simulink model "Cinematica_Inversa (1)"  (R2019a)
settings: Solver=VariableStepAuto  StartTime=0.0  StopTime=10.0  RelTol=1e-3
libraries: arduinolib x6
settings Model: Creator=PATRICIA PEÑALOZA  LastModifiedBy=PATRICIA PEÑALOZA

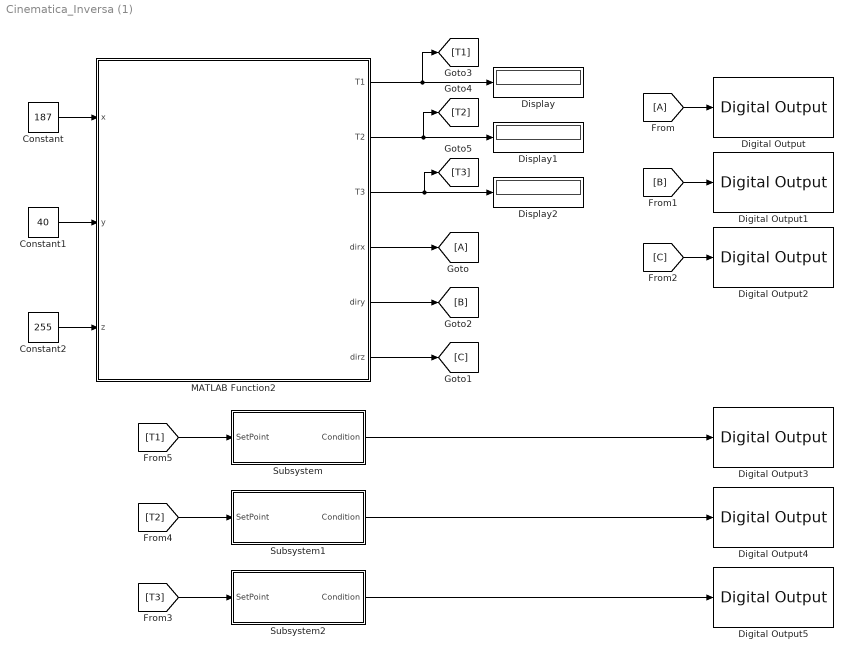
== system Cinematica_Inversa (1) ==
  Constant : Constant  Value=187
  Constant1 : Constant  Value=40
  Constant2 : Constant  Value=255
  Digital Output{,1..5} (6 alike) : arduinolib/Digital Output  pinNumber=9  blockPlatform=arduino
  Display : Display
  Display1 : Display
  Display2 : Display
  MATLAB Function2 : MATLAB Function  TreatAsAtomicUnit=on
  Subsystem : Subsystem
  Subsystem1 : Subsystem
  Subsystem2 : Subsystem
  wires:
  MATLAB Function2/5(diry) -> [B]
  MATLAB Function2/6(dirz) -> [C]
  Constant2/1 -> MATLAB Function2/3(z)
  Subsystem/1(Condition) -> Digital Output3/1
  MATLAB Function2/3(T3) -> [T3], Display2/1
  [T2] -> Subsystem1/1(SetPoint)
  MATLAB Function2/2(T2) -> [T2], Display1/1
  [B] -> Digital Output1/1
  Constant1/1 -> MATLAB Function2/2(y)
  [T3] -> Subsystem2/1(SetPoint)
  [T1] -> Subsystem/1(SetPoint)
  Constant/1 -> MATLAB Function2/1(x)
  [C] -> Digital Output2/1
  Subsystem2/1(Condition) -> Digital Output5/1
  MATLAB Function2/4(dirx) -> [A]
  [A] -> Digital Output/1
  Subsystem1/1(Condition) -> Digital Output4/1
  MATLAB Function2/1(T1) -> [T1], Display/1

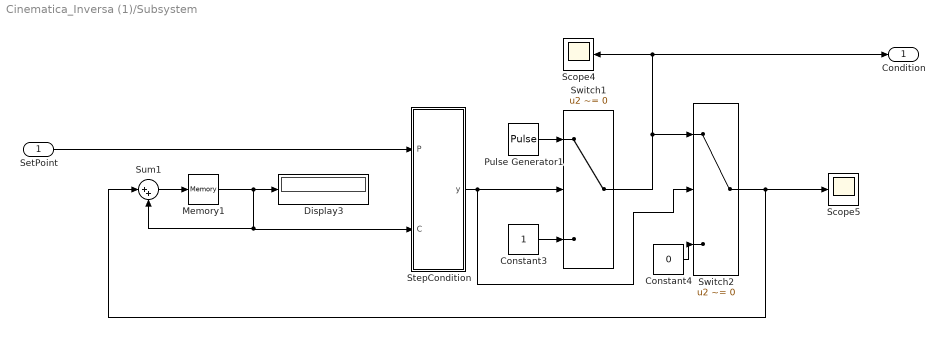
== system Cinematica_Inversa (1)/Subsystem ==
  SetPoint : Inport
  Constant3 : Constant
  Constant4 : Constant  Value=0
  Display3 : Display
  Memory1 : Memory
  Pulse Generator1 : DiscretePulseGenerator  PulseType=Time based  Period=0.0005  PulseWidth=50  PhaseDelay=0.5  VectorParams1D=off
  Scope4 : Scope
  Scope5 : Scope
  StepCondition : MATLAB Function  TreatAsAtomicUnit=on
  Sum1 : Sum  Inputs=|++
  Switch1 : Switch  Criteria=u2 ~= 0
  Switch2 : Switch  Criteria=u2 ~= 0
  Condition : Outport
  wires:
  StepCondition/1(y) -> Switch1/2, Switch2/2
  Memory1/1 -> Display3/1, Sum1/2, StepCondition/2(C)
  Sum1/1 -> Memory1/1
  Switch1/1 -> Scope4/1, Condition/1, Switch2/1
  Constant3/1 -> Switch1/3
  Pulse Generator1/1 -> Switch1/1
  Constant4/1 -> Switch2/3
  SetPoint/1 -> StepCondition/1(P)
  Switch2/1 -> Sum1/1, Scope5/1

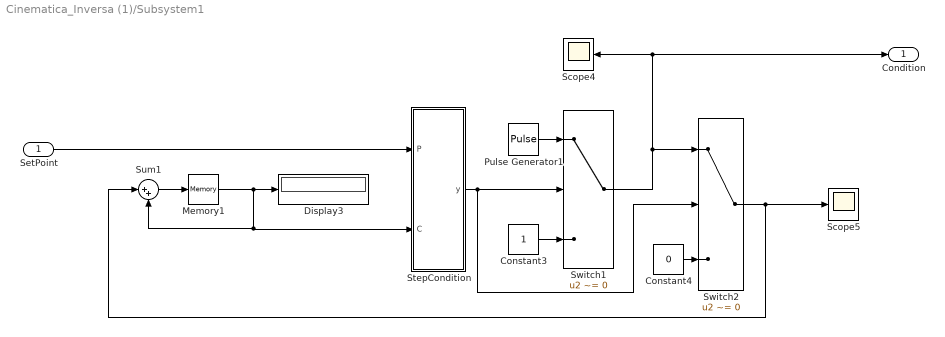
== system Cinematica_Inversa (1)/Subsystem1 ==
  SetPoint : Inport
  Constant3 : Constant
  Constant4 : Constant  Value=0
  Display3 : Display
  Memory1 : Memory
  Pulse Generator1 : DiscretePulseGenerator  PulseType=Time based  Period=0.0005  PulseWidth=50  PhaseDelay=0.5  VectorParams1D=off
  Scope4 : Scope
  Scope5 : Scope
  StepCondition : MATLAB Function  TreatAsAtomicUnit=on
  Sum1 : Sum  Inputs=|++
  Switch1 : Switch  Criteria=u2 ~= 0
  Switch2 : Switch  Criteria=u2 ~= 0
  Condition : Outport
  wires:
  Switch2/1 -> Scope5/1, Sum1/1
  SetPoint/1 -> StepCondition/1(P)
  Constant4/1 -> Switch2/3
  Pulse Generator1/1 -> Switch1/1
  Constant3/1 -> Switch1/3
  Switch1/1 -> Switch2/1, Condition/1, Scope4/1
  Sum1/1 -> Memory1/1
  Memory1/1 -> StepCondition/2(C), Sum1/2, Display3/1
  StepCondition/1(y) -> Switch2/2, Switch1/2

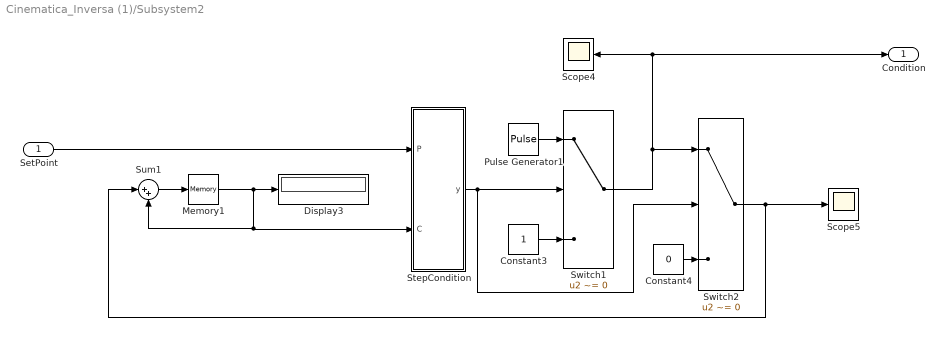
== system Cinematica_Inversa (1)/Subsystem2 ==
  SetPoint : Inport
  Constant3 : Constant
  Constant4 : Constant  Value=0
  Display3 : Display
  Memory1 : Memory
  Pulse Generator1 : DiscretePulseGenerator  PulseType=Time based  Period=0.0005  PulseWidth=50  PhaseDelay=0.5  VectorParams1D=off
  Scope4 : Scope
  Scope5 : Scope
  StepCondition : MATLAB Function  TreatAsAtomicUnit=on
  Sum1 : Sum  Inputs=|++
  Switch1 : Switch  Criteria=u2 ~= 0
  Switch2 : Switch  Criteria=u2 ~= 0
  Condition : Outport
  wires:
  Switch2/1 -> Scope5/1, Sum1/1
  SetPoint/1 -> StepCondition/1(P)
  Constant4/1 -> Switch2/3
  Pulse Generator1/1 -> Switch1/1
  Constant3/1 -> Switch1/3
  Switch1/1 -> Switch2/1, Condition/1, Scope4/1
  Sum1/1 -> Memory1/1
  Memory1/1 -> StepCondition/2(C), Sum1/2, Display3/1
  StepCondition/1(y) -> Switch2/2, Switch1/2

== matlab function Cinematica_Inversa (1)/Subsystem1/StepCondition ==
  data: P input; y output; C input
function y = SC(P,C)
if C==P
    y=0;
else
    y=1;
end

== matlab function Cinematica_Inversa (1)/Subsystem2/StepCondition ==
  data: P input; y output; C input
function y = SC(P,C)
if C==P
    y=0;
else
    y=1;
end

== matlab function Cinematica_Inversa (1)/MATLAB Function2 ==
  data: x input; T1 output; y input; z input; T2 output; T3 output; dirx output; diry output; dirz output
function [T1, T2, T3,dirx, diry, dirz] = Inversa(x, y, z)
l1 = 122; 
l2 = 120;
l3 = 120;
 Tx = atan2d(y,x);
 Dv2 = (x^2 + y^2 + (z - l1)^2 - l2^2 - l3^2)/(2*l2*l3);
 Tz = atan2d(+sqrt(1 - Dv2^2),Dv2);
 Ty = atan2d(z - l1,sqrt(x^2 + y^2)) - atan2d(l3*sind(Tz),l2 + l3*cosd(Tz));
 T1 = round(abs((Tx/1.8)));
 T2 = round(abs(Ty/1.8))
 T3 = abs(round((Tz/1.8)));
 
 if (Tx < 0)
     dirx = 0;
 else
     dirx =1;
 end
     if (Ty < 0)
     diry = 0;
 else
     diry =1;
     end 
     if (Tz < 0)
     dirz = 0;
 else
     dirz =1;
     end 
   
 end

== matlab function Cinematica_Inversa (1)/Subsystem/StepCondition ==
  data: P input; y output; C input
function y = SC(P,C)
if C==P
    y=0;
else
    y=1;
end
